simulink model "v00_0A_0D"  (R2022b)
settings: Solver=FixedStepDiscrete  StartTime=0.0  StopTime=8000  FixedStep=SampleTime  MaxStep=Contactors_StepTime_msec  RelTol=1e-3  EnableMultiTasking=on
undefined symbols (not defined in the file): A_to_mA, BalancingTempGroup, canChannel, CapacityFactor, CC_Inputs, CellSOC, ChargeState, ContactorsFlags, DiscIntNeverNeededParam, gEN_Contactors_StepTime_msec, Ion, isDynamicCurrentEn, Lithium, maxAllowedImbalance, nCells_parallel, nCells_series, nCellTempGrps, PermanentFailRecoveryTrigger, ProtectionFlags, RBal_ohm, SampleTime, sigbuilder_block, StLineEq_varA, StLineEq_varB, TempSelectForDCL, Thresholds, V_to_mV
libraries: simulink x32, spsIdealSwitchLib x21, spsBatteryLib x20, spsSeriesRLCBranchLib x20, spsVoltageMeasurementLib x20, canmsglib x4, canlib x3, dspstat3 x2, spspowerguiLib x2, spsControlledCurrentSourceLib x1, spsCurrentMeasurementLib x1
(part 4 of 7)

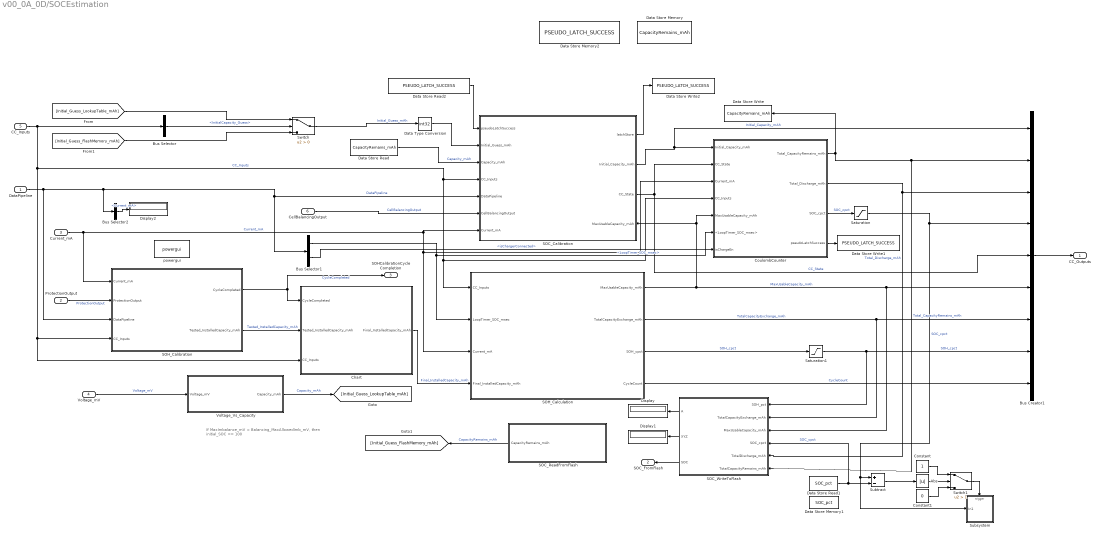
== system v00_0A_0D/SOCEstimation ==
  note: If MaxImbalance_mV < Balancing_MaxAllowedImb_mV, then initial_SOC == 100
  DataPipeline : Inport
  ProtectionOutput : Inport  Port=2
  Current_mA : Inport  Port=3
  Voltage_mV : Inport  Port=4
  CC_Inputs : Inport  Port=5
  CellBalancingOutput : Inport  Port=6
  Abs : Abs  SaturateOnIntegerOverflow=off
  Bus Creator1 : BusCreator  Inputs=9  OutDataTypeStr=Bus: CC_OutputsBus  NonVirtualBus=on
  Bus Selector : BusSelector  OutputSignals=InitialCapacity_Guess
  Bus Selector1 : BusSelector  OutputSignals=LoopTimer_SOC_msec,VCU.isChargerConnected
  Bus Selector2 : BusSelector  OutputSignals=Current_mA
  Chart : Stateflow chart  TreatAsAtomicUnit=on
  Constant : Constant
  Constant1 : Constant  Value=0
  CoulombCounter : Subsystem
  Data Store Memory1 : DataStoreMemory  DataStoreName=SOC_pct  WriteAfterWriteMsg=warning  ShowAdditionalParam=off
  Data Store Memory2 : DataStoreMemory  DataStoreName=PSEUDO_LATCH_SUCCESS  WriteAfterWriteMsg=warning  InitialValue=false  ShowAdditionalParam=off  OutDataTypeStr=boolean
  Data Store Read1 : DataStoreRead  DataStoreName=SOC_pct  IndexOptions=Index vector (dialog)  Indices=1  OutputSizes=1
  Data Store Read2 : DataStoreRead  DataStoreName=PSEUDO_LATCH_SUCCESS  IndexOptions=Index vector (dialog)  Indices=1  OutputSizes=1
  Data Store Write1 : DataStoreWrite  DataStoreName=PSEUDO_LATCH_SUCCESS  IndexOptions=Index vector (dialog)  Indices=1  OutputSizes=1
  Data Store Write2 : DataStoreWrite  DataStoreName=PSEUDO_LATCH_SUCCESS  IndexOptions=Index vector (dialog)  Indices=1  OutputSizes=1
  Data Store Memory : DataStoreMemory  DataStoreName=CapacityRemains_mAh  WriteAfterWriteMsg=warning  ShowAdditionalParam=off
  Data Store Read : DataStoreRead  DataStoreName=CapacityRemains_mAh  IndexOptions=Index vector (dialog)  Indices=1  OutputSizes=1
  Data Store Write : DataStoreWrite  DataStoreName=CapacityRemains_mAh  IndexOptions=Index vector (dialog)  Indices=1  OutputSizes=1
  Data Type Conversion : DataTypeConversion  OutDataTypeStr=int32  SaturateOnIntegerOverflow=off  RndMeth=Floor
  Display : Display
  Display1 : Display
  Display2 : Display
  SOC_Calibration : Subsystem
      settings: PortSchema="{\"entries\":[{\"content\":{\"sides\":[{\"content\":{\"connectorIds\":[\"In1\",\"In2\",\"In3\",\"In4\",\"In5\",\"In6\",\"In7\"]},\"type\":\"ConnectorPlacement.EquallySpacedRectSide\",\"uuid\":\"191a1a7b-14f6-493e-8d18-c1bf9614254a\"},{\"content\":{\"connectorIds\":[\"Out1\",\"Out2\",\"Out3\",\"In8\"],\"side\":\"RIGHT\"},\"type\":\"ConnectorPlacement.EquallySpacedRectSide\",\"uuid\":\"6e4ccf5e-a2af-44ab-8f1a-c43608fc365c\"},{\"content\":{\"connectorIds\":[],\"side\":\"TOP\"},\"type\":\"ConnectorPlacement.EquallySpacedRectSide\",\"uuid\":\"a37c63d5-a375-4ba2-a3db-6b45f5622f96\"}]},\"type\":\"ConnectorPlacement.EquallySpacedConnector\",\"uuid\":\"c93c178a-c38a-42fc-8a0c-0ee2141e96cb\"}],\"packageUris\":[\"http://schema.mathworks.com/mf0/Connector/R2020b\"],\"version\":\"1.0\"}"
  SOC_ReadFromFlash : MATLAB Function  TreatAsAtomicUnit=on  RTWFcnName=VoltagemV_Vs_CapacitymAh
      settings: RTWFcnNameOpts=Use subsystem name  RTWFileNameOpts=Use subsystem name
  SOC_WriteToFlash : MATLAB Function  TreatAsAtomicUnit=on
      settings: RTWFcnNameOpts=Use subsystem name  RTWFileNameOpts=Use subsystem name
  SOH_Calculation : Subsystem
  SOH_Calibration : Subsystem
  Saturation : Saturate  UpperLimit=10000  LowerLimit=0
  Saturation1 : Saturate  UpperLimit=10000  LowerLimit=0
  Subsystem : Subsystem
  Subtract : Sum  Inputs=+-
  Switch : Switch  Criteria=u2 > Threshold  SaturateOnIntegerOverflow=off  InputSameDT=off
  Switch1 : Switch  Criteria=u2 > Threshold  Threshold=1  SaturateOnIntegerOverflow=off  InputSameDT=off
  Voltage_Vs_Capacity : MATLAB Function  TreatAsAtomicUnit=on  RTWFcnName=VoltagemV_Vs_CapacitymAh
      settings: RTWFileNameOpts=Use function name
  powergui : spspowerguiLib/powergui  Priority=1  SimulationMode=Discrete  SampleTime=0.1  frequency=60  Iterations=50  frequencyindice=60  Pbase=100e6  ErrMax=1e-4  UnitsV=kV  UnitsW=MW  buscounter=0  FunctionMessages=off  echomessages=off  EnableUseOfTLC=off  CurrentSourceSwitches=off  DisableSnubberDevices=off  DisableRonSwitches=off  DisableVfSwitches=off  DisplayEquations=off  AutomaticDiscreteSolvers=off  SolverType=Tustin/Backward Euler (TBE)  Interpol=off  ExternalGateDelay=off  methode=off  Ts=100  x0status=blocks  SPID=on  SwTol=0  HookPort=off  NonlinearTolerance=1e-4  nMaxIteration=100  ContinueOnMaxIteration=off  RestoreLinks=warning  ResistiveCurrentMeasurement=off  Frange=[0:2:500]  Ylog=off  Xlog=on  ShowGrid=off  save=off  variable=ZData  structure=0  ZoomFFT=off  StartTime=0.0  cycles=1  DisplayStyle=1  fundamental=60  FreqAxis=off  MaxFrequency=1000  frequencyindicesteady=1  RmsSteady=1  display=off
  CC_Outputs : Outport
  SOC_FromFlash : Outport  Port=2
  SOHCalibrationCycleCompletion : Outport  Port=3
  wires:
  CoulombCounter/2(Total_Discharge_mAh) -> SOC_WriteToFlash/5(TotalDischarge_mAh), Bus Creator1/3  "Total_Discharge_mAh"
  Bus Creator1/1 -> CC_Outputs/1
  CoulombCounter/3(SOC_cpct) -> Saturation/1  "SOC_cpct"
  CoulombCounter/1(Total_CapacityRemains_mAh) -> SOC_WriteToFlash/6(TotalCapacityRemains_mAh), Bus Creator1/2, Data Store Write/1  "Total_CapacityRemains_mAh"
  Voltage_mV/1 -> Voltage_Vs_Capacity/1(Voltage_mV)  "Voltage_mV"
  Voltage_Vs_Capacity/1(Capacity_mAh) -> [Initial_Guess_LookupTable_mAh]  "Capacity_mAh"
  Bus Selector/1 -> Switch/2  "<InitialCapacity_Guess>"
  Switch/1 -> Data Type Conversion/1  "Initial_Guess_mAh"
  [Initial_Guess_LookupTable_mAh] -> Switch/1
  [Initial_Guess_FlashMemory_mAh] -> Switch/3
  SOH_Calculation/1(MaxUsableCapacity_mAh) -> CoulombCounter/5(MaxUsableCapacity_mAh), SOC_Calibration/8(MaxUsableCapacity_mAh), Bus Creator1/6, SOC_WriteToFlash/3(MaxUsableCapacity_mAh)  "MaxUsableCapacity_mAh"
  SOH_Calculation/2(TotalCapacityExchange_mAh) -> Bus Creator1/7, SOC_WriteToFlash/2(TotalCapacityExchange_mAh)  "TotalCapacityExchange_mAh"
  SOH_Calculation/3(SOH_cpct) -> Saturation1/1  "SOH_cpct"
  SOC_ReadFromFlash/1(CapacityRemains_mAh) -> [Initial_Guess_FlashMemory_mAh]  "CapacityRemains_mAh"
  Data Store Read1/1 -> SOC_WriteToFlash/4(SOC_cpct), Subtract/2  "SOC_cpct"
  Subtract/1 -> Abs/1
  Abs/1 -> Switch1/2
  Switch1/1 -> Subsystem/Trigger
  Constant/1 -> Switch1/1
  Constant1/1 -> Switch1/3
  SOH_Calculation/4(CycleCount) -> Bus Creator1/9  "CycleCount"
  SOC_WriteToFlash/3(SOC) -> SOC_FromFlash/1
  Bus Selector1/1 -> SOH_Calculation/2(LoopTimer_SOC_msec), CoulombCounter/6(<LoopTimer_SOC_msec>)  "<LoopTimer_SOC_msec>"
  SOC_WriteToFlash/1(A) -> Display/1
  SOC_WriteToFlash/2(XYZ) -> Display1/1
  Current_mA/1 -> SOC_Calibration/7(Current_mA), CoulombCounter/3(Current_mA), SOH_Calculation/3(Current_mA), SOH_Calibration/1(Current_mA)  "Current_mA"
  ProtectionOutput/1 -> SOH_Calibration/2(ProtectionOutput)  "ProtectionOutput"
  CC_Inputs/1 -> Bus Selector/1, SOH_Calculation/1(CC_Inputs), CoulombCounter/4(CC_Inputs), SOC_Calibration/4(CC_Inputs), Chart/3(CC_Inputs), SOH_Calibration/4(CC_Inputs)  "CC_Inputs"
  DataPipeline/1 -> Bus Selector2/1, Bus Selector1/1, SOC_Calibration/5(DataPipeline), SOH_Calibration/3(DataPipeline)  "DataPipeline"
  Chart/1(Final_InstalledCapacity_mAh) -> SOH_Calculation/4(Final_InstalledCapacity_mAh)  "Final_InstalledCapacity_mAh"
  SOH_Calibration/2(Tested_InstalledCapacity_mAh) -> Chart/2(Tested_InstalledCapacity_mAh)  "Tested_InstalledCapacity_mAh"
  SOH_Calibration/1(CycleCompleted) -> SOHCalibrationCycleCompletion/1, Chart/1(CycleCompleted)  "CycleCompleted"
  Saturation/1 -> Subtract/1, Subsystem/1(In1), Bus Creator1/4  "SOC_cpct"
  Saturation1/1 -> Bus Creator1/8, SOC_WriteToFlash/1(SOH_pct)  "SOH_cpct"
  SOC_Calibration/3(CC_State) -> CoulombCounter/2(CC_State), Bus Creator1/5  "CC_State"
  SOC_Calibration/2(Initial_Capacity_mAh) -> Bus Creator1/1, CoulombCounter/1(Initial_Capacity_mAh)  "Initial_Capacity_mAh"
  Data Type Conversion/1 -> SOC_Calibration/2(Initial_Guess_mAh)
  CellBalancingOutput/1 -> SOC_Calibration/6(CellBalancingOutput)  "CellBalancingOutput"
  Data Store Read/1 -> SOC_Calibration/3(Capacity_mAh)  "Capacity_mAh"
  Bus Selector2/1 -> Display2/1  "<Current_mA>"
  Bus Selector1/2 -> CoulombCounter/7(isChargeEn)  "<isChargerConnected>"
  CoulombCounter/4(pseudoLatchSuccess) -> Data Store Write1/1
  Data Store Read2/1 -> SOC_Calibration/1(pseudoLatchSuccess)
  SOC_Calibration/1(latchStore) -> Data Store Write2/1

== system v00_0A_0D/Signal Builder ==
  Demux : Demux  Tag=STV Demux  Outputs=1
      settings: DisplayOption=none
  FromWs : FromWorkspace  Tag=STV FromWs  VariableName=tuvar  SampleTime=0.1
      SigBuilderData=|
      | common.afterFinalStr = 'Extrapolate'
      | common.sampleTime = '0.1'
      | dataSet.timeRange = [1 4013]
      | dataSet.name = 'Sheet1'
      | sbobj.Groups.Name = 'Sheet1'
      | sbobj.Groups.Signals.Name = 'Out'
      | sbobj.Groups.Signals.XData = [1 2 3 4 5 6 7 8 9 10 11 12 ... (4013 elements, 1x4013)]
      | sbobj.Groups.Signals.YData = [100 100 100 100 100 100 100 100 100 100 100 100 ... (4013 elements, 1x4013)]
      | sbobj.Groups.TimeRange = [1 4013]
  Out : Outport  Tag=STV Outport
  wires:
  Demux/1 -> Out/1
  FromWs/1 -> Demux/1

== system v00_0A_0D/Signal Builder1 ==
  Demux : Demux  Tag=STV Demux  Outputs=1
      settings: DisplayOption=none
  FromWs : FromWorkspace  Tag=STV FromWs  VariableName=tuvar  SampleTime=0.1
      SigBuilderData=|
      | common.afterFinalStr = 'Extrapolate'
      | common.sampleTime = '0.1'
      | dataSet.timeRange = [0 4000.7]
      | dataSet.name = 'Group 1'
      | sbobj.Groups.Name = 'Group 1'
      | sbobj.Groups.Signals.Name = 'Signal 1'
      | sbobj.Groups.Signals.XData = [0 1670 2590 4000.7]
      | sbobj.Groups.Signals.YData = [200 200 200 200]
      | sbobj.Groups.TimeRange = [0 4000.7]
  Signal 1 : Outport  Tag=STV Outport
  wires:
  Demux/1 -> Signal 1/1
  FromWs/1 -> Demux/1

== system v00_0A_0D/Signal Builder2 ==
  Demux : Demux  Tag=STV Demux  Outputs=1
      settings: DisplayOption=none
  FromWs : FromWorkspace  Tag=STV FromWs  VariableName=tuvar  SampleTime=0.1
      SigBuilderData=|
      | common.afterFinalStr = 'Extrapolate'
      | common.sampleTime = '0.1'
      | dataSet.timeRange = [0 4000.7]
      | dataSet.name = 'Group 1'
      | sbobj.Groups.Name = 'Group 1'
      | sbobj.Groups.Signals.Name = 'Signal 1'
      | sbobj.Groups.Signals.XData = [0 1670 2590 4000.7]
      | sbobj.Groups.Signals.YData = [0 0 0 0]
      | sbobj.Groups.TimeRange = [0 4000.7]
  Signal 1 : Outport  Tag=STV Outport
  wires:
  FromWs/1 -> Demux/1
  Demux/1 -> Signal 1/1

== system v00_0A_0D/Signal Builder3 ==
  Demux : Demux  Tag=STV Demux  Outputs=1
      settings: DisplayOption=none
  FromWs : FromWorkspace  Tag=STV FromWs  VariableName=tuvar  SampleTime=0.1
      SigBuilderData=|
      | common.afterFinalStr = 'Extrapolate'
      | common.sampleTime = '0.1'
      | dataSet.timeRange = [0 4000.7]
      | dataSet.name = 'Group 1'
      | sbobj.Groups.Name = 'Group 1'
      | sbobj.Groups.Signals.Name = 'Signal 1'
      | sbobj.Groups.Signals.XData = [0 1670 2200 4000.7]
      | sbobj.Groups.Signals.YData = [500 400 300 200]
      | sbobj.Groups.TimeRange = [0 4000.7]
  Signal 1 : Outport  Tag=STV Outport
  wires:
  Demux/1 -> Signal 1/1
  FromWs/1 -> Demux/1

== system v00_0A_0D/Cell Blocks1/Signal Builder ==
  Demux : Demux  Tag=STV Demux  Outputs=1
      settings: DisplayOption=none
  FromWs : FromWorkspace  Tag=STV FromWs  VariableName=tuvar
      SigBuilderData=|
      | common.afterFinalStr = 'Extrapolate'
      | common.sampleTime = 0
      | dataSet.timeRange = [0 4000]
      | dataSet.name = 'Group 1'
      | sbobj.Groups.Name = 'Group 1'
      | sbobj.Groups.Signals.Name = 'Signal 1'
      | sbobj.Groups.Signals.XData = [0 100 100 1500 3000 4000]
      | sbobj.Groups.Signals.YData = [23.15 24.25 24.2 32.85 27 22.7]
      | sbobj.Groups.TimeRange = [0 4000]
  Signal 1 : Outport  Tag=STV Outport
  wires:
  Demux/1 -> Signal 1/1
  FromWs/1 -> Demux/1

== system v00_0A_0D/Cell Blocks1/Signal Builder1 ==
  Demux : Demux  Tag=STV Demux  Outputs=1
      settings: DisplayOption=none
  FromWs : FromWorkspace  Tag=STV FromWs  VariableName=tuvar
      SigBuilderData=|
      | common.afterFinalStr = 'Extrapolate'
      | common.sampleTime = 0
      | dataSet.timeRange = [0 4000]
      | dataSet.name = 'Group 1'
      | sbobj.Groups.Name = 'Group 1'
      | sbobj.Groups.Signals.Name = 'Signal 1'
      | sbobj.Groups.Signals.XData = [0 100 1500 3000 4000]
      | sbobj.Groups.Signals.YData = [26 25.9 26.5 26 26.85]
      | sbobj.Groups.TimeRange = [0 4000]
  Signal 1 : Outport  Tag=STV Outport
  wires:
  FromWs/1 -> Demux/1
  Demux/1 -> Signal 1/1

== system v00_0A_0D/Cell Blocks1/Signal Builder10 ==
  Demux : Demux  Tag=STV Demux  Outputs=1
      settings: DisplayOption=none
  FromWs : FromWorkspace  Tag=STV FromWs  VariableName=tuvar
      SigBuilderData=|
      | common.afterFinalStr = 'Extrapolate'
      | common.sampleTime = 0
      | dataSet.timeRange = [0 4000]
      | dataSet.name = 'Group 1'
      | sbobj.Groups.Name = 'Group 1'
      | sbobj.Groups.Signals.Name = 'Signal 1'
      | sbobj.Groups.Signals.XData = [0 100 1500 3000 4000]
      | sbobj.Groups.Signals.YData = [26 25.9 26.5 26 26.85]
      | sbobj.Groups.TimeRange = [0 4000]
  Signal 1 : Outport  Tag=STV Outport
  wires:
  FromWs/1 -> Demux/1
  Demux/1 -> Signal 1/1

== system v00_0A_0D/Cell Blocks1/Signal Builder11 ==
  Demux : Demux  Tag=STV Demux  Outputs=1
      settings: DisplayOption=none
  FromWs : FromWorkspace  Tag=STV FromWs  VariableName=tuvar
      SigBuilderData=|
      | common.afterFinalStr = 'Extrapolate'
      | common.sampleTime = 0
      | dataSet.timeRange = [0 4000]
      | dataSet.name = 'Group 1'
      | sbobj.Groups.Name = 'Group 1'
      | sbobj.Groups.Signals.Name = 'Signal 1'
      | sbobj.Groups.Signals.XData = [0 100 1500 3000 4000]
      | sbobj.Groups.Signals.YData = [26 25.9 26.5 26 26.85]
      | sbobj.Groups.TimeRange = [0 4000]
  Signal 1 : Outport  Tag=STV Outport
  wires:
  Demux/1 -> Signal 1/1
  FromWs/1 -> Demux/1

== system v00_0A_0D/Cell Blocks1/Signal Builder12 ==
  Demux : Demux  Tag=STV Demux  Outputs=1
      settings: DisplayOption=none
  FromWs : FromWorkspace  Tag=STV FromWs  VariableName=tuvar
      SigBuilderData=|
      | common.afterFinalStr = 'Extrapolate'
      | common.sampleTime = 0
      | dataSet.timeRange = [0 4000]
      | dataSet.name = 'Group 1'
      | sbobj.Groups.Name = 'Group 1'
      | sbobj.Groups.Signals.Name = 'Signal 1'
      | sbobj.Groups.Signals.XData = [0 100 1500 3000 4000]
      | sbobj.Groups.Signals.YData = [26 25.9 26.5 26 26.85]
      | sbobj.Groups.TimeRange = [0 4000]
  Signal 1 : Outport  Tag=STV Outport
  wires:
  FromWs/1 -> Demux/1
  Demux/1 -> Signal 1/1

== system v00_0A_0D/Cell Blocks1/Signal Builder13 ==
  Demux : Demux  Tag=STV Demux  Outputs=1
      settings: DisplayOption=none
  FromWs : FromWorkspace  Tag=STV FromWs  VariableName=tuvar
      SigBuilderData=|
      | common.afterFinalStr = 'Extrapolate'
      | common.sampleTime = 0
      | dataSet.timeRange = [0 4000]
      | dataSet.name = 'Group 1'
      | sbobj.Groups.Name = 'Group 1'
      | sbobj.Groups.Signals.Name = 'Signal 1'
      | sbobj.Groups.Signals.XData = [0 100 1500 3000 4000]
      | sbobj.Groups.Signals.YData = [26 25.9 26.5 26 26.85]
      | sbobj.Groups.TimeRange = [0 4000]
  Signal 1 : Outport  Tag=STV Outport
  wires:
  Demux/1 -> Signal 1/1
  FromWs/1 -> Demux/1

== system v00_0A_0D/Cell Blocks1/Signal Builder14 ==
  Demux : Demux  Tag=STV Demux  Outputs=1
      settings: DisplayOption=none
  FromWs : FromWorkspace  Tag=STV FromWs  VariableName=tuvar
      SigBuilderData=|
      | common.afterFinalStr = 'Extrapolate'
      | common.sampleTime = 0
      | dataSet.timeRange = [0 4000]
      | dataSet.name = 'Group 1'
      | sbobj.Groups.Name = 'Group 1'
      | sbobj.Groups.Signals.Name = 'Signal 1'
      | sbobj.Groups.Signals.XData = [0 100 1500 3000 4000]
      | sbobj.Groups.Signals.YData = [26 25.9 26.5 26 26.85]
      | sbobj.Groups.TimeRange = [0 4000]
  Signal 1 : Outport  Tag=STV Outport
  wires:
  Demux/1 -> Signal 1/1
  FromWs/1 -> Demux/1

== system v00_0A_0D/Cell Blocks1/Signal Builder2 ==
  Demux : Demux  Tag=STV Demux  Outputs=1
      settings: DisplayOption=none
  FromWs : FromWorkspace  Tag=STV FromWs  VariableName=tuvar
      SigBuilderData=|
      | common.afterFinalStr = 'Extrapolate'
      | common.sampleTime = 0
      | dataSet.timeRange = [0 4000]
      | dataSet.name = 'Group 1'
      | sbobj.Groups.Name = 'Group 1'
      | sbobj.Groups.Signals.Name = 'Signal 1'
      | sbobj.Groups.Signals.XData = [0 300 1000 1500 4000]
      | sbobj.Groups.Signals.YData = [188500 188500 -180000 188000 12000]
      | sbobj.Groups.TimeRange = [0 4000]
  Signal 1 : Outport  Tag=STV Outport
  wires:
  Demux/1 -> Signal 1/1
  FromWs/1 -> Demux/1

== system v00_0A_0D/Cell Blocks1/Signal Builder3 ==
  Demux : Demux  Tag=STV Demux  Outputs=1
      settings: DisplayOption=none
  FromWs : FromWorkspace  Tag=STV FromWs  VariableName=tuvar
      SigBuilderData=|
      | common.afterFinalStr = 'Extrapolate'
      | common.sampleTime = 0
      | dataSet.timeRange = [0 4000]
      | dataSet.name = 'Group 1'
      | sbobj.Groups.Name = 'Group 1'
      | sbobj.Groups.Signals.Name = 'Signal 1'
      | sbobj.Groups.Signals.XData = [0 100 1500 3000 4000]
      | sbobj.Groups.Signals.YData = [26 25.9 26.5 26 26.85]
      | sbobj.Groups.TimeRange = [0 4000]
  Signal 1 : Outport  Tag=STV Outport
  wires:
  Demux/1 -> Signal 1/1
  FromWs/1 -> Demux/1

== system v00_0A_0D/Cell Blocks1/Signal Builder4 ==
  Demux : Demux  Tag=STV Demux  Outputs=1
      settings: DisplayOption=none
  FromWs : FromWorkspace  Tag=STV FromWs  VariableName=tuvar
      SigBuilderData=|
      | common.afterFinalStr = 'Extrapolate'
      | common.sampleTime = 0
      | dataSet.timeRange = [0 4000]
      | dataSet.name = 'Group 1'
      | sbobj.Groups.Name = 'Group 1'
      | sbobj.Groups.Signals.Name = 'Signal 1'
      | sbobj.Groups.Signals.XData = [0 100 1500 3000 4000]
      | sbobj.Groups.Signals.YData = [26 25.9 26.5 26 26.85]
      | sbobj.Groups.TimeRange = [0 4000]
  Signal 1 : Outport  Tag=STV Outport
  wires:
  FromWs/1 -> Demux/1
  Demux/1 -> Signal 1/1

== system v00_0A_0D/Cell Blocks1/Signal Builder5 ==
  Demux : Demux  Tag=STV Demux  Outputs=1
      settings: DisplayOption=none
  FromWs : FromWorkspace  Tag=STV FromWs  VariableName=tuvar
      SigBuilderData=|
      | common.afterFinalStr = 'Extrapolate'
      | common.sampleTime = 0
      | dataSet.timeRange = [0 4000]
      | dataSet.name = 'Group 1'
      | sbobj.Groups.Name = 'Group 1'
      | sbobj.Groups.Signals.Name = 'Signal 1'
      | sbobj.Groups.Signals.XData = [0 100 1500 3000 4000]
      | sbobj.Groups.Signals.YData = [26 25.9 26.5 26 26.85]
      | sbobj.Groups.TimeRange = [0 4000]
  Signal 1 : Outport  Tag=STV Outport
  wires:
  Demux/1 -> Signal 1/1
  FromWs/1 -> Demux/1

== system v00_0A_0D/Cell Blocks1/Signal Builder6 ==
  Demux : Demux  Tag=STV Demux  Outputs=1
      settings: DisplayOption=none
  FromWs : FromWorkspace  Tag=STV FromWs  VariableName=tuvar
      SigBuilderData=|
      | common.afterFinalStr = 'Extrapolate'
      | common.sampleTime = 0
      | dataSet.timeRange = [0 4000]
      | dataSet.name = 'Group 1'
      | sbobj.Groups.Name = 'Group 1'
      | sbobj.Groups.Signals.Name = 'Signal 1'
      | sbobj.Groups.Signals.XData = [0 100 1500 3000 4000]
      | sbobj.Groups.Signals.YData = [26 25.9 26.5 26 26.85]
      | sbobj.Groups.TimeRange = [0 4000]
  Signal 1 : Outport  Tag=STV Outport
  wires:
  FromWs/1 -> Demux/1
  Demux/1 -> Signal 1/1

== system v00_0A_0D/Cell Blocks1/Signal Builder7 ==
  Demux : Demux  Tag=STV Demux  Outputs=1
      settings: DisplayOption=none
  FromWs : FromWorkspace  Tag=STV FromWs  VariableName=tuvar
      SigBuilderData=|
      | common.afterFinalStr = 'Extrapolate'
      | common.sampleTime = 0
      | dataSet.timeRange = [0 4000]
      | dataSet.name = 'Group 1'
      | sbobj.Groups.Name = 'Group 1'
      | sbobj.Groups.Signals.Name = 'Signal 1'
      | sbobj.Groups.Signals.XData = [0 100 1500 3000 4000]
      | sbobj.Groups.Signals.YData = [26 25.9 26.5 26 26.85]
      | sbobj.Groups.TimeRange = [0 4000]
  Signal 1 : Outport  Tag=STV Outport
  wires:
  Demux/1 -> Signal 1/1
  FromWs/1 -> Demux/1

== system v00_0A_0D/Cell Blocks1/Signal Builder8 ==
  Demux : Demux  Tag=STV Demux  Outputs=1
      settings: DisplayOption=none
  FromWs : FromWorkspace  Tag=STV FromWs  VariableName=tuvar
      SigBuilderData=|
      | common.afterFinalStr = 'Extrapolate'
      | common.sampleTime = 0
      | dataSet.timeRange = [0 4000]
      | dataSet.name = 'Group 1'
      | sbobj.Groups.Name = 'Group 1'
      | sbobj.Groups.Signals.Name = 'Signal 1'
      | sbobj.Groups.Signals.XData = [0 100 1500 3000 4000]
      | sbobj.Groups.Signals.YData = [26 25.9 26.5 26 26.85]
      | sbobj.Groups.TimeRange = [0 4000]
  Signal 1 : Outport  Tag=STV Outport
  wires:
  FromWs/1 -> Demux/1
  Demux/1 -> Signal 1/1

== system v00_0A_0D/Cell Blocks1/Signal Builder9 ==
  Demux : Demux  Tag=STV Demux  Outputs=1
      settings: DisplayOption=none
  FromWs : FromWorkspace  Tag=STV FromWs  VariableName=tuvar
      SigBuilderData=|
      | common.afterFinalStr = 'Extrapolate'
      | common.sampleTime = 0
      | dataSet.timeRange = [0 4000]
      | dataSet.name = 'Group 1'
      | sbobj.Groups.Name = 'Group 1'
      | sbobj.Groups.Signals.Name = 'Signal 1'
      | sbobj.Groups.Signals.XData = [0 100 1500 3000 4000]
      | sbobj.Groups.Signals.YData = [26 25.9 26.5 26 26.85]
      | sbobj.Groups.TimeRange = [0 4000]
  Signal 1 : Outport  Tag=STV Outport
  wires:
  Demux/1 -> Signal 1/1
  FromWs/1 -> Demux/1

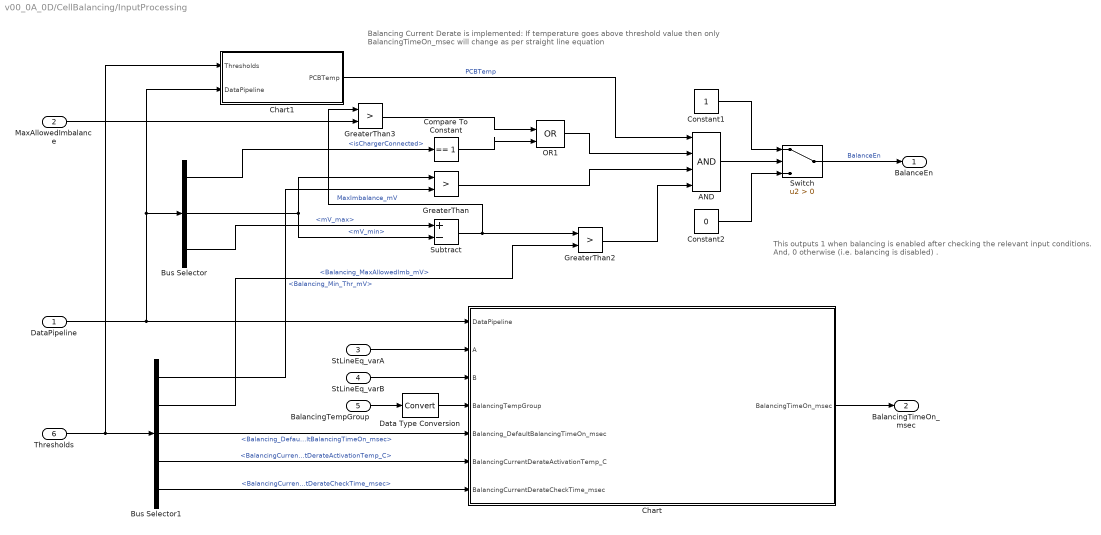
== system v00_0A_0D/CellBalancing/InputProcessing ==
  note: Balancing Current Derate is implemented: If temperature goes above threshold value then only BalancingTimeOn_msec will change as per straight line equation
  note: This outputs 1 when balancing is enabled
      | after checking the relevant input conditions.
      | And, 0 otherwise (i.e. balancing is disabled) .
  DataPipeline : Inport
  MaxAllowedImbalance : Inport  Port=2
  StLineEq_varA : Inport  Port=3
  StLineEq_varB : Inport  Port=4
  BalancingTempGroup : Inport  Port=5
  Thresholds : Inport  Port=6
  AND : Logic  Inputs=4  IconShape=distinctive  AllPortsSameDT=off  OutDataTypeStr=boolean
  Bus Selector : BusSelector  OutputSignals=VCU.isChargerConnected,VoltageSenseBus.mV_min,VoltageSenseBus.mV_max
  Bus Selector1 : BusSelector  OutputSignals=Balancing_Min_Thr_mV,Balancing_MaxAllowedImb_mV,Balancing_DefaultBalancingTimeOn_msec,BalancingCurrentDerateActivationTemp_C,BalancingCurrentDerateCheckTime_msec
  Chart : Stateflow chart  TreatAsAtomicUnit=on
  Chart1 : Stateflow chart  TreatAsAtomicUnit=on
  Compare To Constant : simulink/Logic and Bit Operations/Compare To Constant  relop===  const=1  OutDataTypeStr=boolean
  Constant1 : Constant  OutDataTypeStr=boolean
  Constant2 : Constant  Value=0  OutDataTypeStr=boolean
  Data Type Conversion : DataTypeConversion  SaturateOnIntegerOverflow=off  RndMeth=Floor
  GreaterThan : RelationalOperator  Operator=>  OutDataTypeStr=boolean  RndMeth=Simplest  InputSameDT=off
  GreaterThan2 : RelationalOperator  Operator=>  OutDataTypeStr=boolean  RndMeth=Simplest  InputSameDT=off
  GreaterThan3 : RelationalOperator  Operator=>  OutDataTypeStr=boolean  RndMeth=Simplest  InputSameDT=off
  OR1 : Logic  Operator=OR  IconShape=distinctive  AllPortsSameDT=off  OutDataTypeStr=boolean
  Subtract : Sum  Inputs=+-
  Switch : Switch  Criteria=u2 > Threshold  OutDataTypeStr=boolean  SaturateOnIntegerOverflow=off  InputSameDT=off
  BalanceEn : Outport
  BalancingTimeOn_msec : Outport  Port=2
  wires:
  Bus Selector/3 -> Subtract/1  "<mV_max>"
  Bus Selector/1 -> Compare To Constant/1  "<isChargerConnected>"
  Bus Selector/2 -> GreaterThan/1, Subtract/2  "<mV_min>"
  Bus Selector1/1 -> GreaterThan/2  "<Balancing_Min_Thr_mV>"
  Compare To Constant/1 -> OR1/2
  AND/1 -> Switch/2
  Constant1/1 -> Switch/1
  Constant2/1 -> Switch/3
  Subtract/1 -> GreaterThan2/1, GreaterThan3/1  "MaxImbalance_mV"
  BalancingTempGroup/1 -> Data Type Conversion/1
  StLineEq_varB/1 -> Chart/3(B)
  StLineEq_varA/1 -> Chart/2(A)
  DataPipeline/1 -> Chart/1(DataPipeline), Chart1/2(DataPipeline), Bus Selector/1
  Chart/1(BalancingTimeOn_msec) -> BalancingTimeOn_msec/1
  Switch/1 -> BalanceEn/1  "BalanceEn"
  GreaterThan2/1 -> AND/4
  GreaterThan/1 -> AND/3
  OR1/1 -> AND/2
  Thresholds/1 -> Chart1/1(Thresholds), Bus Selector1/1
  Bus Selector1/2 -> GreaterThan2/2  "<Balancing_MaxAllowedImb_mV>"
  Bus Selector1/3 -> Chart/5(Balancing_DefaultBalancingTimeOn_msec)  "<Balancing_DefaultBalancingTimeOn_msec>"
  Bus Selector1/4 -> Chart/6(BalancingCurrentDerateActivationTemp_C)  "<BalancingCurrentDerateActivationTemp_C>"
  Bus Selector1/5 -> Chart/7(BalancingCurrentDerateCheckTime_msec)  "<BalancingCurrentDerateCheckTime_msec>"
  Chart1/1(PCBTemp) -> AND/1  "PCBTemp"
  Data Type Conversion/1 -> Chart/4(BalancingTempGroup)
  MaxAllowedImbalance/1 -> GreaterThan3/2
  GreaterThan3/1 -> OR1/1

== system v00_0A_0D/DataPipeline/GetN3 ==
  Array : Inport
  NArray : Outport
  wires:
  Array/1 -> NArray/1

== system v00_0A_0D/HeartbeatMonitoring_Initial/Enabled Subsystem ==
  Enable : EnablePort
  Add : Sum
  Constant : Constant  Value=0.1  OutDataTypeStr=single
  Unit Delay : UnitDelay  SampleTime=-1  HasFrameUpgradeWarning=on
  Out1 : Outport
  wires:
  Unit Delay/1 -> Add/2
  Add/1 -> Out1/1, Unit Delay/1
  Constant/1 -> Add/1

== system v00_0A_0D/HeartbeatMonitoring_Initial/Signal Builder ==
  Demux : Demux  Tag=STV Demux  Outputs=1
      settings: DisplayOption=none
  FromWs : FromWorkspace  Tag=STV FromWs  VariableName=tuvar
      SigBuilderData=|
      | common.afterFinalStr = 'Extrapolate'
      | common.sampleTime = 0
      | dataSet.timeRange = [0 4000.7]
      | dataSet.name = 'Group 1'
      | sbobj.Groups.Name = 'Group 1'
      | sbobj.Groups.Signals.Name = 'Signal 1'
      | sbobj.Groups.Signals.XData = [0 2500 2500 3000 3000 4000.7]
      | sbobj.Groups.Signals.YData = [0.995 1 0 0 1 1]
      | sbobj.Groups.TimeRange = [0 4000.7]
  Signal 1 : Outport  Tag=STV Outport
  wires:
  FromWs/1 -> Demux/1
  Demux/1 -> Signal 1/1

== system v00_0A_0D/Protection/Triggered Subsystem ==
  Now_Tmax : Inport
  Now_mV_min : Inport  Port=2
  Trigger : TriggerPort  VariantControl=(inherit)
  Old_Tmax : Outport
  Old_mV_min : Outport  Port=2
  wires:
  Now_Tmax/1 -> Old_Tmax/1
  Now_mV_min/1 -> Old_mV_min/1

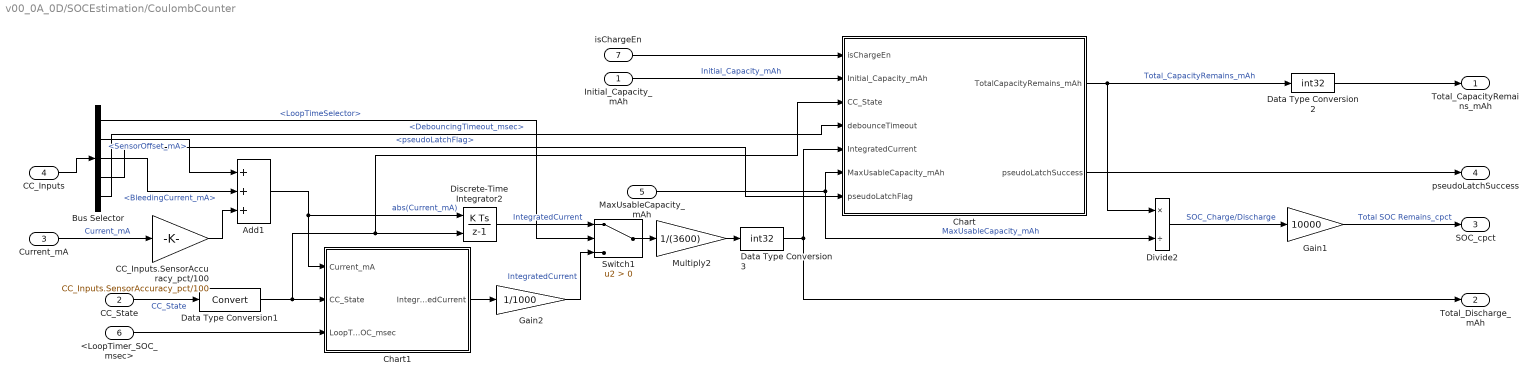
== system v00_0A_0D/SOCEstimation/CoulombCounter ==
  Initial_Capacity_mAh : Inport
  CC_State : Inport  Port=2
  Current_mA : Inport  Port=3
  CC_Inputs : Inport  Port=4
  MaxUsableCapacity_mAh : Inport  Port=5
  <LoopTimer_SOC_msec> : Inport  Port=6
  isChargeEn : Inport  Port=7
  Add1 : Sum  Inputs=+++
  Bus Selector : BusSelector  OutputSignals=LoopTimeSelector,SensorOffset_mA,BleedingCurrent_mA,pseudoLatchFlag,DebouncingTimeout_msec
  CC_Inputs.SensorAccuracy_pct/100 : Gain  Gain=CC_Inputs.SensorAccuracy_pct/100  OutDataTypeStr=single
  Chart : Stateflow chart  TreatAsAtomicUnit=on
  Chart1 : Stateflow chart  TreatAsAtomicUnit=on
      settings: PortSchema="{\"entries\":[{\"content\":{\"sides\":[{\"content\":{\"connectorIds\":[\"In2\",\"In3\",\"In1\"]},\"type\":\"ConnectorPlacement.EquallySpacedRectSide\",\"uuid\":\"e2992fff-d326-494d-90ab-e8ab9b17f1b1\"},{\"content\":{\"connectorIds\":[\"Out1\"],\"side\":\"RIGHT\"},\"type\":\"ConnectorPlacement.EquallySpacedRectSide\",\"uuid\":\"bbfd7a6e-6fa6-46b0-8c55-f4f0467cd268\"},{\"content\":{\"connectorIds\":[],\"side\":\"TOP\"},\"type\":\"ConnectorPlacement.EquallySpacedRectSide\",\"uuid\":\"defcbc16-e3da-481e-a98a-d33339a1314b\"},{\"content\":{\"connectorIds\":[],\"side\":\"BOTTOM\"},\"type\":\"ConnectorPlacement.EquallySpacedRectSide\",\"uuid\":\"01077edb-bafc-47ec-abcb-be5cab7dbb10\"}]},\"type\":\"ConnectorPlacement.EquallySpacedConnector\",\"uuid\":\"f3897327-e846-46f2-83ec-430392605691\"}],\"packageUris\":[\"http://schema.mathworks.com/mf0/Connector/R2020b\"],\"version\":\"1.0\"}"
  Data Type Conversion1 : DataTypeConversion  SaturateOnIntegerOverflow=off  RndMeth=Floor
  Data Type Conversion2 : DataTypeConversion  OutDataTypeStr=int32  SaturateOnIntegerOverflow=off  RndMeth=Floor
  Data Type Conversion3 : DataTypeConversion  OutDataTypeStr=int32  SaturateOnIntegerOverflow=off  RndMeth=Floor
  Discrete-Time Integrator2 : DiscreteIntegrator  ExternalReset=rising  SampleTime=SampleTime  ICPrevOutput=DiscIntNeverNeededParam  ICPrevScaledInput=DiscIntNeverNeededParam
  Divide2 : Product  Inputs=*/  OutDataTypeStr=double
  Gain1 : Gain  Gain=10000  OutDataTypeStr=int32
  Gain2 : Gain  Gain=1/1000
  Multiply2 : Gain  Gain=1/(3600)  OutDataTypeStr=single
  Switch1 : Switch  Criteria=u2 > Threshold  SaturateOnIntegerOverflow=off  InputSameDT=off
  Total_CapacityRemains_mAh : Outport
  Total_Discharge_mAh : Outport  Port=2
  SOC_cpct : Outport  Port=3
  pseudoLatchSuccess : Outport  Port=4
  wires:
  Chart1/1(IntegratedCurrent) -> Gain2/1
  Bus Selector/1 -> Switch1/2  "<LoopTimeSelector>"
  Discrete-Time Integrator2/1 -> Switch1/1  "IntegratedCurrent"
  Add1/1 -> Chart1/2(Current_mA), Discrete-Time Integrator2/1  "abs(Current_mA)"
  Current_mA/1 -> CC_Inputs.SensorAccuracy_pct/100/1  "Current_mA"
  Initial_Capacity_mAh/1 -> Chart/2(Initial_Capacity_mAh)  "Initial_Capacity_mAh"
  CC_Inputs.SensorAccuracy_pct/100/1 -> Add1/3
  Data Type Conversion1/1 -> Discrete-Time Integrator2/2, Chart/3(CC_State), Chart1/3(CC_State)
  MaxUsableCapacity_mAh/1 -> Chart/6(MaxUsableCapacity_mAh), Divide2/2  "MaxUsableCapacity_mAh"
  CC_State/1 -> Data Type Conversion1/1  "CC_State"
  Switch1/1 -> Multiply2/1
  Divide2/1 -> Gain1/1  "SOC_Charge/Discharge"
  Gain1/1 -> SOC_cpct/1  "Total SOC Remains_cpct"
  Data Type Conversion2/1 -> Total_CapacityRemains_mAh/1
  Gain2/1 -> Switch1/3  "IntegratedCurrent"
  CC_Inputs/1 -> Bus Selector/1
  Bus Selector/2 -> Add1/1  "<SensorOffset_mA>"
  Bus Selector/3 -> Add1/2  "<BleedingCurrent_mA>"
  Data Type Conversion3/1 -> Chart/5(IntegratedCurrent), Total_Discharge_mAh/1
  Chart/1(TotalCapacityRemains_mAh) -> Divide2/1, Data Type Conversion2/1  "Total_CapacityRemains_mAh"
  <LoopTimer_SOC_msec>/1 -> Chart1/1(LoopTimer_SOC_msec)
  isChargeEn/1 -> Chart/1(isChargeEn)
  Multiply2/1 -> Data Type Conversion3/1
  Bus Selector/4 -> Chart/7(pseudoLatchFlag)  "<pseudoLatchFlag>"
  Chart/2(pseudoLatchSuccess) -> pseudoLatchSuccess/1
  Bus Selector/5 -> Chart/4(debounceTimeout)  "<DebouncingTimeout_msec>"

== system v00_0A_0D/SOCEstimation/SOC_Calibration ==
  pseudoLatchSuccess : Inport
  Initial_Guess_mAh : Inport  Port=2
  Capacity_mAh : Inport  Port=3
  CC_Inputs : Inport  Port=4
  DataPipeline : Inport  Port=5
  CellBalancingOutput : Inport  Port=6
  Current_mA : Inport  Port=7
  MaxUsableCapacity_mAh : Inport  Port=8
  Bus Selector : BusSelector  OutputSignals=minVoltageForLatch_mV,FastCharge.MaxAllowedImb_mV,SlowCharge.MaxAllowedImb_mV,FastCharge.MaxCurrentLimit_mA,SlowCharge.MaxCurrentLimit_mA,FastCharge.MinCurrentLimit_mA,SlowCharge.MinCurrentLimit_mA,DebouncingTimeout_msec
  Bus Selector1 : BusSelector  OutputSignals=VCU.FastCharge
  SOC_Calibration : Stateflow chart  TreatAsAtomicUnit=on
      settings: PortSchema="{\"entries\":[{\"content\":{\"sides\":[{\"content\":{\"connectorIds\":[\"In3\",\"In8\",\"In4\",\"In2\",\"In7\",\"In6\",\"In5\",\"In9\",\"In10\",\"In11\",\"In1\",\"In12\",\"In13\"]},\"type\":\"ConnectorPlacement.EquallySpacedRectSide\",\"uuid\":\"b3b2fd03-86cb-4726-8fd8-0cf60b090956\"},{\"content\":{\"connectorIds\":[\"Out3\",\"Out2\",\"Out1\"],\"side\":\"RIGHT\"},\"type\":\"ConnectorPlacement.EquallySpacedRectSide\",\"uuid\":\"4b3699fd-923a-4261-9ecd-9e3cbe0d64e5\"},{\"content\":{\"connectorIds\":[],\"side\":\"TOP\"},\"type\":\"ConnectorPlacement.EquallySpacedRectSide\",\"uuid\":\"7532a1c1-253b-462b-bb47-60ab9f5bddde\"},{\"content\":{\"connectorIds\":[],\"side\":\"BOTTOM\"},\"type\":\"ConnectorPlacement.EquallySpacedRectSide\",\"uuid\":\"5ce0e271-f51a-40da-9bd6-9edac805e4b7\"}]},\"type\":\"ConnectorPlacement.EquallySpacedConnector\",\"uuid\":\"34f487d6-2367-443a-a7f3-b057a6a8eb7a\"}],\"packageUris\":[\"http://schema.mathworks.com/mf0/Connector/R2020b\"],\"version\":\"1.0\"}"
  Switch1 : Switch  Criteria=u2 > Threshold  SaturateOnIntegerOverflow=off  InputSameDT=off
  Switch2 : Switch  Criteria=u2 > Threshold  SaturateOnIntegerOverflow=off  InputSameDT=off
  Switch3 : Switch  Criteria=u2 > Threshold  SaturateOnIntegerOverflow=off  InputSameDT=off
  latchStore : Outport
  Initial_Capacity_mAh : Outport  Port=2
  CC_State : Outport  Port=3
  wires:
  MaxUsableCapacity_mAh/1 -> SOC_Calibration/2(MaxUsableCapacity_mAh)  "MaxUsableCapacity_mAh"
  CC_Inputs/1 -> SOC_Calibration/5(CC_Inputs), Bus Selector/1
  Initial_Guess_mAh/1 -> SOC_Calibration/3(Initial_Guess_mAh)  "Initial_Guess_mAh"
  CellBalancingOutput/1 -> SOC_Calibration/7(CellBalancingOutput)  "CellBalancingOutput"
  Capacity_mAh/1 -> SOC_Calibration/8(Capacity_mAh)  "Capacity_mAh"
  SOC_Calibration/1(CC_State) -> CC_State/1  "CC_State"
  SOC_Calibration/3(Initial_Capacity_mAh) -> Initial_Capacity_mAh/1  "Initial_Capacity_mAh"
  Current_mA/1 -> SOC_Calibration/4(Current_mA)  "Current_mA"
  DataPipeline/1 -> SOC_Calibration/6(DataPipeline), Bus Selector1/1  "DataPipeline"
  Bus Selector1/1 -> Switch3/2, Switch2/2, Switch1/2  "<FastCharge>"
  Switch1/1 -> SOC_Calibration/10(MaxAllowedImb_mV)  "MaxAllowedImb_mV"
  Switch2/1 -> SOC_Calibration/11(MaxCurrentLimit_mA)  "MaxCurrentLimit_mA"
  Switch3/1 -> SOC_Calibration/1(MinCurrentLimit_mA)  "MinCurrentLimit_mA"
  Bus Selector/2 -> Switch1/1  "<MaxAllowedImb_mV>"
  Bus Selector/3 -> Switch1/3  "<MaxAllowedImb_mV>"
  Bus Selector/4 -> Switch2/1  "<MaxCurrentLimit_mA>"
  Bus Selector/5 -> Switch2/3  "<MaxCurrentLimit_mA>"
  Bus Selector/6 -> Switch3/1  "<MinCurrentLimit_mA>"
  Bus Selector/7 -> Switch3/3  "<MinCurrentLimit_mA>"
  Bus Selector/8 -> SOC_Calibration/12(DebouncingTimeout_msec)  "<DebouncingTimeout_msec>"
  Bus Selector/1 -> SOC_Calibration/9(minVoltageForLatch)  "<minVoltageForLatch_mV>"
  pseudoLatchSuccess/1 -> SOC_Calibration/13("pseudoLatchSuccess ")
  SOC_Calibration/2(pseudoLatchSuccess) -> latchStore/1

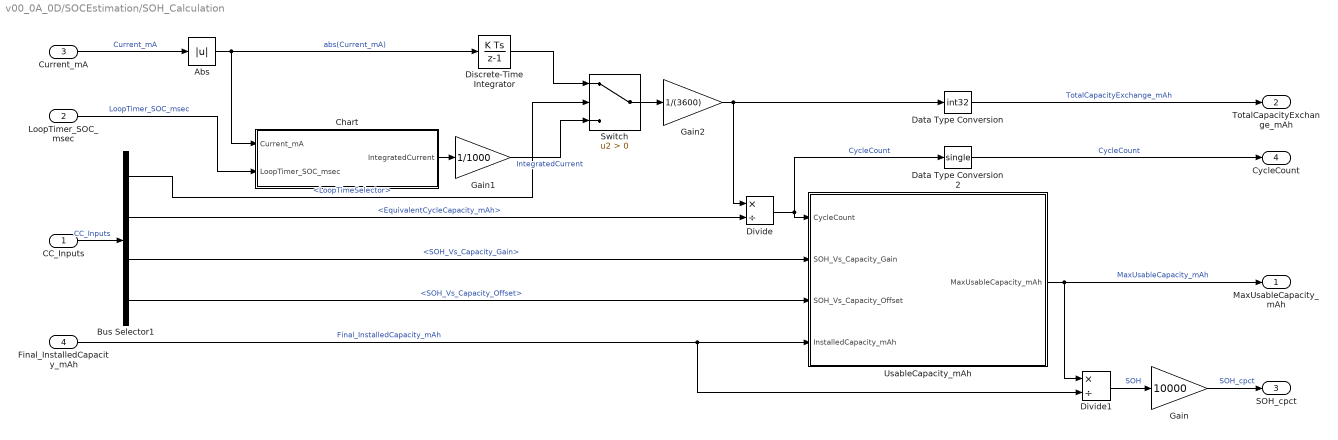
== system v00_0A_0D/SOCEstimation/SOH_Calculation ==
  CC_Inputs : Inport
  LoopTimer_SOC_msec : Inport  Port=2
  Current_mA : Inport  Port=3
  Final_InstalledCapacity_mAh : Inport  Port=4
  Abs : Abs  SaturateOnIntegerOverflow=off
  Bus Selector1 : BusSelector  OutputSignals=LoopTimeSelector,EquivalentCycleCapacity_mAh,SOH_Vs_Capacity_Gain,SOH_Vs_Capacity_Offset
  Chart : Stateflow chart  TreatAsAtomicUnit=on
      settings: PortSchema="{\"entries\":[{\"content\":{\"sides\":[{\"content\":{\"connectorIds\":[\"In2\",\"In1\"]},\"type\":\"ConnectorPlacement.EquallySpacedRectSide\",\"uuid\":\"fa2b1eb4-ea10-4b58-a108-6883031cdbb9\"},{\"content\":{\"connectorIds\":[\"Out1\"],\"side\":\"RIGHT\"},\"type\":\"ConnectorPlacement.EquallySpacedRectSide\",\"uuid\":\"771b5087-a593-4bec-8ae0-d1d746b48b0a\"},{\"content\":{\"connectorIds\":[],\"side\":\"TOP\"},\"type\":\"ConnectorPlacement.EquallySpacedRectSide\",\"uuid\":\"93c5daf7-1610-4016-b338-8118b9847b6e\"}]},\"type\":\"ConnectorPlacement.EquallySpacedConnector\",\"uuid\":\"693d00d1-3a85-40b4-83e9-189846b81cab\"}],\"packageUris\":[\"http://schema.mathworks.com/mf0/Connector/R2020b\"],\"version\":\"1.0\"}"
  Data Type Conversion : DataTypeConversion  OutDataTypeStr=int32  SaturateOnIntegerOverflow=off  RndMeth=Floor
  Data Type Conversion2 : DataTypeConversion  OutDataTypeStr=single  SaturateOnIntegerOverflow=off  RndMeth=Floor
  Discrete-Time Integrator : DiscreteIntegrator  SampleTime=SampleTime  OutDataTypeStr=single  ICPrevOutput=DiscIntNeverNeededParam  ICPrevScaledInput=DiscIntNeverNeededParam
  Divide : Product  Inputs=*/  OutDataTypeStr=single
  Divide1 : Product  Inputs=*/  OutDataTypeStr=single
  Gain : Gain  Gain=10000  OutDataTypeStr=int32
  Gain1 : Gain  Gain=1/1000
  Gain2 : Gain  Gain=1/(3600)  OutDataTypeStr=single
  Switch : Switch  Criteria=u2 > Threshold  SaturateOnIntegerOverflow=off  InputSameDT=off
  UsableCapacity_mAh : MATLAB Function  TreatAsAtomicUnit=on
      settings: RTWFcnNameOpts=Use subsystem name  RTWFileNameOpts=Use subsystem name
  MaxUsableCapacity_mAh : Outport
  TotalCapacityExchange_mAh : Outport  Port=2
  SOH_cpct : Outport  Port=3
  CycleCount : Outport  Port=4
  wires:
  Current_mA/1 -> Abs/1  "Current_mA"
  Abs/1 -> Discrete-Time Integrator/1, Chart/2(Current_mA)  "abs(Current_mA)"
  Divide/1 -> UsableCapacity_mAh/1(CycleCount), Data Type Conversion2/1  "CycleCount"
  UsableCapacity_mAh/1(MaxUsableCapacity_mAh) -> MaxUsableCapacity_mAh/1, Divide1/1  "MaxUsableCapacity_mAh"
  Divide1/1 -> Gain/1  "SOH"
  Gain/1 -> SOH_cpct/1  "SOH_cpct"
  Bus Selector1/3 -> UsableCapacity_mAh/2(SOH_Vs_Capacity_Gain)  "<SOH_Vs_Capacity_Gain>"
  Bus Selector1/4 -> UsableCapacity_mAh/3(SOH_Vs_Capacity_Offset)  "<SOH_Vs_Capacity_Offset>"
  Data Type Conversion2/1 -> CycleCount/1  "CycleCount"
  Data Type Conversion/1 -> TotalCapacityExchange_mAh/1  "TotalCapacityExchange_mAh"
  Gain2/1 -> Data Type Conversion/1, Divide/1
  LoopTimer_SOC_msec/1 -> Chart/1(LoopTimer_SOC_msec)  "LoopTimer_SOC_msec"
  Switch/1 -> Gain2/1
  Chart/1(IntegratedCurrent) -> Gain1/1
  Discrete-Time Integrator/1 -> Switch/1
  Gain1/1 -> Switch/3  "IntegratedCurrent"
  CC_Inputs/1 -> Bus Selector1/1  "CC_Inputs"
  Bus Selector1/2 -> Divide/2  "<EquivalentCycleCapacity_mAh>"
  Bus Selector1/1 -> Switch/2  "<LoopTimeSelector>"
  Final_InstalledCapacity_mAh/1 -> Divide1/2, UsableCapacity_mAh/4(InstalledCapacity_mAh)  "Final_InstalledCapacity_mAh"

== system v00_0A_0D/SOCEstimation/SOH_Calibration ==
  Current_mA : Inport
  ProtectionOutput : Inport  Port=2
  DataPipeline : Inport  Port=3
  CC_Inputs : Inport  Port=4
  Bus Selector : BusSelector  OutputSignals=LoopTimer_SOC_msec
  SOH_Calibration : Stateflow chart  TreatAsAtomicUnit=on
  Subsystem : Subsystem
  CycleCompleted : Outport
  Tested_InstalledCapacity_mAh : Outport  Port=2
  wires:
  Current_mA/1 -> Subsystem/2(Current_mA)  "Current_mA"
  SOH_Calibration/1(CalcEnable) -> Subsystem/Enable  "CalcEnable"
  SOH_Calibration/2(CycleCompleted) -> CycleCompleted/1, Subsystem/1(CycleCompleted)  "CycleCompleted"
  DataPipeline/1 -> Bus Selector/1, SOH_Calibration/3(DataPipeline)  "DataPipeline"
  ProtectionOutput/1 -> SOH_Calibration/1(ProtectionOutput)  "ProtectionOutput"
  CC_Inputs/1 -> SOH_Calibration/2(CC_Inputs), Subsystem/4(CC_Inputs)  "CC_Inputs"
  Bus Selector/1 -> Subsystem/3(LoopTimer_SOC_msec)  "<LoopTimer_SOC_msec>"
  Subsystem/1(Tested_InstalledCapacity_mAh) -> Tested_InstalledCapacity_mAh/1  "Tested_InstalledCapacity_mAh"

== system v00_0A_0D/SOCEstimation/Subsystem ==
  In1 : Inport
  Trigger : TriggerPort  VariantControl=(inherit)  PortDimensions=1
  Data Store Write1 : DataStoreWrite  DataStoreName=SOC_pct  DataStoreElements=SOC_pct  IndexOptions=Index vector (dialog)  Indices=1  OutputSizes=1
  wires:
  In1/1 -> Data Store Write1/1

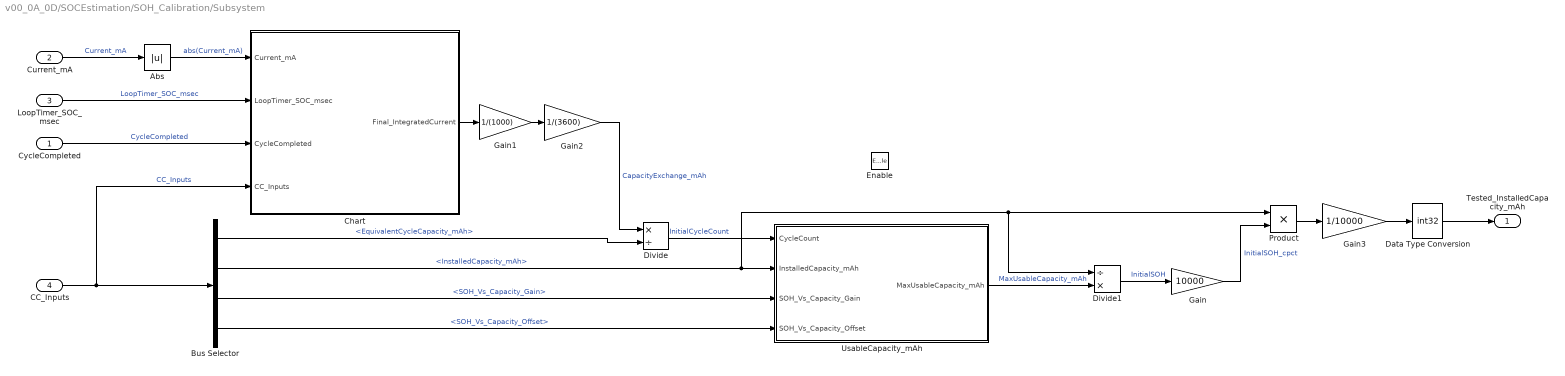
== system v00_0A_0D/SOCEstimation/SOH_Calibration/Subsystem ==
  CycleCompleted : Inport
  Current_mA : Inport  Port=2
  LoopTimer_SOC_msec : Inport  Port=3
  CC_Inputs : Inport  Port=4
  Enable : EnablePort
  Abs : Abs  SaturateOnIntegerOverflow=off
  Bus Selector : BusSelector  OutputSignals=EquivalentCycleCapacity_mAh,InstalledCapacity_mAh,SOH_Vs_Capacity_Gain,SOH_Vs_Capacity_Offset
  Chart : Stateflow chart  TreatAsAtomicUnit=on
      settings: PortSchema="{\"entries\":[{\"content\":{\"sides\":[{\"content\":{\"connectorIds\":[\"In2\",\"In1\",\"In3\",\"In4\"]},\"type\":\"ConnectorPlacement.EquallySpacedRectSide\",\"uuid\":\"fa2b1eb4-ea10-4b58-a108-6883031cdbb9\"},{\"content\":{\"connectorIds\":[\"Out1\"],\"side\":\"RIGHT\"},\"type\":\"ConnectorPlacement.EquallySpacedRectSide\",\"uuid\":\"771b5087-a593-4bec-8ae0-d1d746b48b0a\"},{\"content\":{\"connectorIds\":[],\"side\":\"TOP\"},\"type\":\"ConnectorPlacement.EquallySpacedRectSide\",\"uuid\":\"93c5daf7-1610-4016-b338-8118b9847b6e\"}]},\"type\":\"ConnectorPlacement.EquallySpacedConnector\",\"uuid\":\"693d00d1-3a85-40b4-83e9-189846b81cab\"}],\"packageUris\":[\"http://schema.mathworks.com/mf0/Connector/R2020b\"],\"version\":\"1.0\"}"
  Data Type Conversion : DataTypeConversion  OutDataTypeStr=int32  SaturateOnIntegerOverflow=off  RndMeth=Floor
  Divide : Product  Inputs=*/  OutDataTypeStr=single
  Divide1 : Product  Inputs=/*  OutDataTypeStr=single
  Gain : Gain  Gain=10000  OutDataTypeStr=int32
  Gain1 : Gain  Gain=1/(1000)
  Gain2 : Gain  Gain=1/(3600)  OutDataTypeStr=single
  Gain3 : Gain  Gain=1/10000  OutDataTypeStr=single
  Product : Product  OutDataTypeStr=int32
  UsableCapacity_mAh : MATLAB Function  TreatAsAtomicUnit=on
      settings: RTWFcnNameOpts=Use subsystem name  RTWFileNameOpts=Use subsystem name
  Tested_InstalledCapacity_mAh : Outport
  wires:
  Current_mA/1 -> Abs/1  "Current_mA"
  Gain1/1 -> Gain2/1
  Gain2/1 -> Divide/1  "CapacityExchange_mAh"
  Chart/1(Final_IntegratedCurrent) -> Gain1/1
  Abs/1 -> Chart/2(Current_mA)  "abs(Current_mA)"
  Divide/1 -> UsableCapacity_mAh/1(CycleCount)  "InitialCycleCount"
  LoopTimer_SOC_msec/1 -> Chart/1(LoopTimer_SOC_msec)  "LoopTimer_SOC_msec"
  CycleCompleted/1 -> Chart/3(CycleCompleted)  "CycleCompleted"
  Divide1/1 -> Gain/1  "InitialSOH"
  Gain/1 -> Product/2  "InitialSOH_cpct"
  CC_Inputs/1 -> Bus Selector/1, Chart/4(CC_Inputs)  "CC_Inputs"
  Bus Selector/1 -> Divide/2  "<EquivalentCycleCapacity_mAh>"
  Bus Selector/2 -> UsableCapacity_mAh/2(InstalledCapacity_mAh), Product/1, Divide1/1  "<InstalledCapacity_mAh>"
  Bus Selector/3 -> UsableCapacity_mAh/3(SOH_Vs_Capacity_Gain)  "<SOH_Vs_Capacity_Gain>"
  Bus Selector/4 -> UsableCapacity_mAh/4(SOH_Vs_Capacity_Offset)  "<SOH_Vs_Capacity_Offset>"
  Product/1 -> Gain3/1
  Gain3/1 -> Data Type Conversion/1
  Data Type Conversion/1 -> Tested_InstalledCapacity_mAh/1
  UsableCapacity_mAh/1(MaxUsableCapacity_mAh) -> Divide1/2  "MaxUsableCapacity_mAh"
